simulink model "ECE371_Lab9_part1"  (R2017a)
settings: Solver=ode3  StartTime=0.0  StopTime=25  FixedStep=0.01  RelTol=1e-3
libraries: simulink x4
settings Model: Creator=localmgr  LastModifiedBy=localmgr

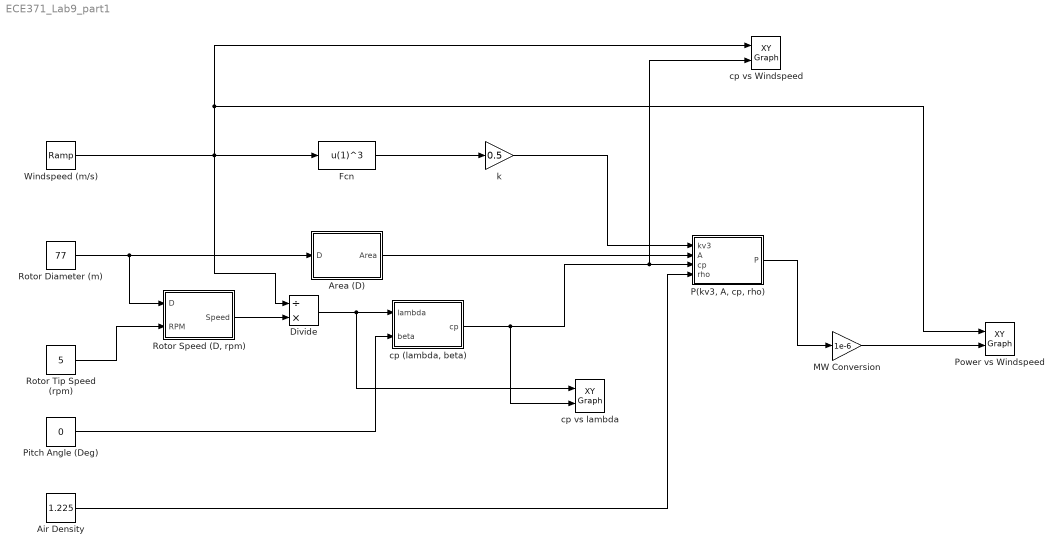
== system ECE371_Lab9_part1 ==
  Air Density : Constant  Value=1.225
  Area (D) : MATLAB Function  TreatAsAtomicUnit=on
  Divide : Product  Inputs=/*
  Fcn : Fcn  Expr=u(1)^3
  MW Conversion : Gain  Gain=1e-6
  "P(kv3, A, cp, rho)" : MATLAB Function  TreatAsAtomicUnit=on
  Pitch Angle (Deg) : Constant  Value=0
  Power vs Windspeed : simulink/Sinks/XY Graph  xmin=0  xmax=25  ymin=0  ymax=0.4  st=0.01
  Rotor Diameter (m) : Constant  Value=77
  "Rotor Speed (D, rpm)" : MATLAB Function  TreatAsAtomicUnit=on
  Rotor Tip Speed (rpm) : Constant  Value=5
  Windspeed (m/s) : simulink/Sources/Ramp  slope=1  start=0  X0=0
  "cp (lambda, beta)" : MATLAB Function  TreatAsAtomicUnit=on
  cp vs Windspeed : simulink/Sinks/XY Graph  xmin=0  xmax=25  ymin=0  ymax=1  st=0.01
  cp vs lambda : simulink/Sinks/XY Graph  xmin=0  xmax=15  ymin=0  ymax=0.5  st=0.01
  k : Gain  Gain=0.5
  wires:
  Rotor Diameter (m)/1 -> "Rotor Speed (D, rpm)"/1(D), Area (D)/1(D)
  Rotor Tip Speed (rpm)/1 -> "Rotor Speed (D, rpm)"/2(RPM)
  Air Density/1 -> "P(kv3, A, cp, rho)"/4(rho)
  "P(kv3, A, cp, rho)"/1(P) -> MW Conversion/1
  MW Conversion/1 -> Power vs Windspeed/2
  "Rotor Speed (D, rpm)"/1(Speed) -> Divide/2
  Windspeed (m/s)/1 -> Divide/1, Power vs Windspeed/1, cp vs Windspeed/1, Fcn/1
  Fcn/1 -> k/1
  k/1 -> "P(kv3, A, cp, rho)"/1(kv3)
  Area (D)/1(Area) -> "P(kv3, A, cp, rho)"/2(A)
  "cp (lambda, beta)"/1(cp) -> cp vs lambda/2, cp vs Windspeed/2, "P(kv3, A, cp, rho)"/3(cp)
  Divide/1 -> cp vs lambda/1, "cp (lambda, beta)"/1(lambda)
  Pitch Angle (Deg)/1 -> "cp (lambda, beta)"/2(beta)

== matlab function ECE371_Lab9_part1/Rotor Speed (D, rpm) ==
  data: D input; Speed output; RPM input
function Speed = fcn(D, RPM)

Speed = RPM*3.14159*D/60;

== matlab function ECE371_Lab9_part1/cp (lambda, beta) ==
  data: lambda input; cp output; beta input
function cp = fcn(lambda, beta)

c1 = 0.52;
c2 = 116;
c3 = 0.4;
c4 = 5;
c5 = 21;
c6 = 0.0068;
lambda_rec = 1/(lambda + 0.08*beta) - 0.035/(beta^3 + 1);

cp = c1*(c2*lambda_rec - c3*beta - c4)*exp(-c5*lambda_rec) + c6*lambda;

== matlab function ECE371_Lab9_part1/P(kv3, A, cp, rho) ==
  data: kv3 input; P output; A input; cp input; rho input
function P = fcn(kv3, A, cp, rho)

P = kv3 * rho * A * cp;

== matlab function ECE371_Lab9_part1/Area (D) ==
  data: D input; Area output
function Area = fcn(D)

Area = 3.14159*D^2/4;
